simulink model "SineWaveTrojectory"  (R2024b)
settings: Solver=FixedStepAuto  StartTime=0.0  StopTime=20  FixedStep=0.05  RelTol=1e-3
values from neighbouring files (symbols this model uses):
  L = 0.5    [SimRun.m]
  R = 0.1    [SimRun.m]
undefined symbols (not defined in the file or in its folder): A, B, C, D, IC
libraries: simulink x1
settings Model: Creator=elija  LastModifiedBy=elija

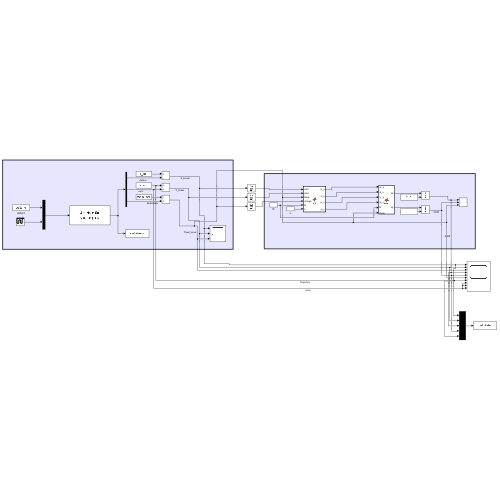
[thumbnail: Simulink's stored preview of the top-level diagram]
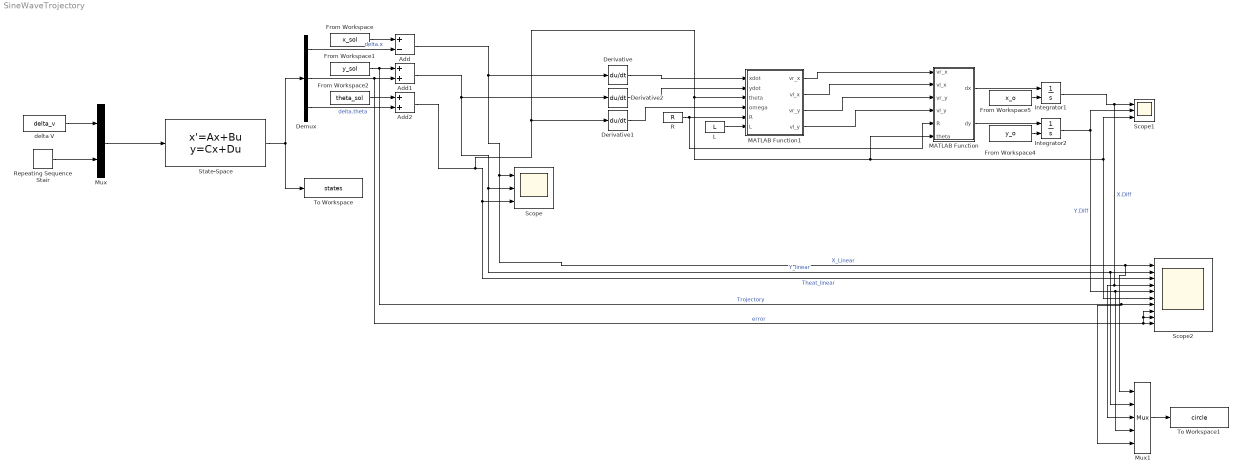
== system SineWaveTrojectory ==
  Add : Sum  Inputs=+-
  Add1 : Sum
  Add2 : Sum
  Demux : Demux  Outputs=3
  Derivative : Derivative
  Derivative1 : Derivative
  Derivative2 : Derivative
  From Workspace : FromWorkspace  VariableName=x_sol
  From Workspace1 : FromWorkspace  VariableName=y_sol
  From Workspace2 : FromWorkspace  VariableName=theta_sol
  From Workspace4 : FromWorkspace  VariableName=y_o
  From Workspace5 : FromWorkspace  VariableName=x_o
  Integrator1 : Integrator  InitialConditionSource=external
  Integrator2 : Integrator  InitialConditionSource=external
  L : Constant  Value=L
  MATLAB Function : MATLAB Function  TreatAsAtomicUnit=on
  MATLAB Function1 : MATLAB Function  TreatAsAtomicUnit=on
  Mux : Mux  Inputs=2
  Mux1 : Mux  Inputs=5
  R : Constant  Value=R
  Repeating Sequence Stair : simulink/Sources/Repeating Sequence Stair  OutValues=[-3*5 -1*5 -3*5 0].'  tsamp=0.5  OutMin=[]  OutMax=[]  OutDataTypeStr=double  OutputDataTypeScalingMode=double  OutDataType=fixdt(0,8)  ConRadixGroup=Best Precision: Vector-wise  OutScaling=2^-12
  Scope : Scope  NumInputPorts=3
  Scope1 : Scope  NumInputPorts=3
  Scope2 : Scope  NumInputPorts=10
  State-Space : StateSpace  A=A  B=B  C=C  D=D  InitialCondition=IC
  To Workspace : ToWorkspace  VariableName=states  SaveFormat=Timeseries  SampleTime=-1
  To Workspace1 : ToWorkspace  VariableName=circle  SaveFormat=Timeseries  SampleTime=-1
  delta V : FromWorkspace  VariableName=delta_v
  wires:
  L/1 -> MATLAB Function1/6(L)
  MATLAB Function1/3(vr_y) -> MATLAB Function/3(vr_y)
  MATLAB Function1/4(vl_y) -> MATLAB Function/4(vl_y)
  Add1/1 -> Mux1/2, Scope2/2, Scope/2, Derivative2/1  "Y_linear"
  R/1 -> MATLAB Function1/5(R), MATLAB Function/5(R)
  From Workspace/1 -> Add/1
  Add2/1 -> Derivative1/1, Scope1/3, Scope2/6, MATLAB Function/6(theta), MATLAB Function1/3(theta), Scope2/3, Scope/3  "Theat_linear"
  Add/1 -> Mux1/1, Scope2/1, Scope/1, Derivative/1  "X_Linear"
  Derivative1/1 -> MATLAB Function1/4(omega)
  Demux/3 -> Add2/2  "delta.theta"
  From Workspace5/1 -> Integrator1/2
  MATLAB Function/2(dy) -> Integrator2/1
  MATLAB Function/1(dx) -> Integrator1/1
  Integrator2/1 -> Scope1/2, Mux1/4, Scope2/5  "Y.Diff"
  Derivative/1 -> MATLAB Function1/1(xdot)
  State-Space/1 -> To Workspace/1, Demux/1
  MATLAB Function1/2(vl_x) -> MATLAB Function/2(vl_x)
  MATLAB Function1/1(vr_x) -> MATLAB Function/1(vr_x)
  delta V/1 -> Mux/1
  Mux/1 -> State-Space/1
  From Workspace1/1 -> Mux1/5, Scope2/7, Add1/1  "Trojectory"
  Demux/2 -> Scope2/8, Scope2/9, Scope2/10, Add1/2  "error"
  Derivative2/1 -> MATLAB Function1/2(ydot)
  From Workspace4/1 -> Integrator2/2
  Demux/1 -> Add/2  "delta.x"
  Integrator1/1 -> Scope1/1, Scope2/4, Mux1/3  "X.Diff"
  From Workspace2/1 -> Add2/1
  Repeating Sequence Stair/1 -> Mux/2
  Mux1/1 -> To Workspace1/1

== matlab function SineWaveTrojectory/MATLAB Function ==
  data: dx output; dy output; vr_x input; vl_x input; vr_y input; vl_y input; R input; theta input
function [dx,dy] = fcn(vr_x,vl_x,vr_y,vl_y,R,theta)

dx = (R./2).*(vr_x+vl_x).*cos(theta);


dy = (R./2).*(vr_y+vl_y).*cos(theta);



end

== matlab function SineWaveTrojectory/MATLAB Function1 ==
  data: xdot input; ydot input; vr_x output; theta input; omega input; R input; vl_x output; L input; vr_y output; vl_y output
function [vr_x,vl_x,vr_y,vl_y] = fcn(xdot,ydot,theta,omega,R,L)

vx = xdot./cos(theta);
vr_x = (2.*vx+omega*L)/(2*R);
vl_x = (2.*vx-omega*L)/(2*R);

vy = ydot./cos(theta);
vr_y = (2.*vy+omega*L)/(2*R);
vl_y = (2.*vy-omega*L)/(2*R);
end
